simulink model "UIO_example"  (R2019b)
settings: Solver=VariableStepAuto  StartTime=0.0  StopTime=30  RelTol=1e-3
values from neighbouring files (symbols this model uses):
  A = [0 1;-5+Lx -4+epsilon*Lx]    [DAC_UIO_Comp.m]    (also in LinearND_QUANTUM_2020_11_14_2.m = A+(basis{i}*rand()); UIO_adaptive_example.m = [-2379.2 0 0 0 0;0 -2.3 0 0.21 0; UIO_adaptive_example_2.m = [-1/Ta, (alpha+sigma2*wb2)/Ta, (-kb*sigma2*wb2)/Ta, -kb*sigm; UIO_adaptive_example_EEG_Balas_2ch.m)
  B1 = [0;0;0;kq*wa^2]    [UIO_adaptive_example.m]    (also in UIO_adaptive_example_2.m)
  B2 = [68245 0 0;0 -2 0;0 0 2;0 232.75 0; 0 0 -232.75]    [UIO_adaptive_example.m]    (also in UIO_adaptive_example_2.m = [1;0;1;0]; UIO_adaptive_example_EEG.m = ones(opt_order,1); UIO_adaptive_example_EEG_Balas_2ch.m = ones(opt_order,1); UIO_adaptive_example_EEG_ch2.m = ones(opt_order,1))
  C = [1, epsilon]    [DAC_UIO_Comp.m]    (also in UIO_adaptive_example.m = [1 0 0 0 0;0 0 0 1 0; 0 0 0 0 1]; UIO_adaptive_example_2.m = [1 0 0 0;0 1 0 0]; UIO_adaptive_example_EEG_Balas_2ch.m; UIO_adaptive_example_alternative_EEG_ch6.m = ss_c.C)
  F = B2'*P/(C)    [UIO_adaptive_example_2.m]    (also in UIO_adaptive_example_EEG.m = B2'*P/(C_data{opt_order}); UIO_adaptive_example_EEG_ch2.m = B2'*P/(C_data{opt_order}); UIO_adaptive_example_EEG_ch2_DEAP.m = B2'*P/(C_data{opt_order}); UIO_adaptive_example_EEG_ch2_ECEO.m = B2'*P/(C_data{opt_order}))
  Gamma = 20    [UIO_adaptive_example_2.m]    (also in UIO_adaptive_example_EEG.m = 0.001; UIO_adaptive_example_EEG_ch2.m = loop(i); UIO_adaptive_example_EEG_ch2_DEAP.m = loop(i); UIO_adaptive_example_EEG_ch2_ECEO.m = loop(i))
  L = inv(P)*Y    [UIO_adaptive_example.m]    (also in UIO_adaptive_example_2.m; UIO_adaptive_example_EEG.m; UIO_adaptive_example_EEG_ch2.m; UIO_adaptive_example_EEG_ch2_DEAP.m)
settings Model: Creator=Tris  LastModifiedBy=Tris

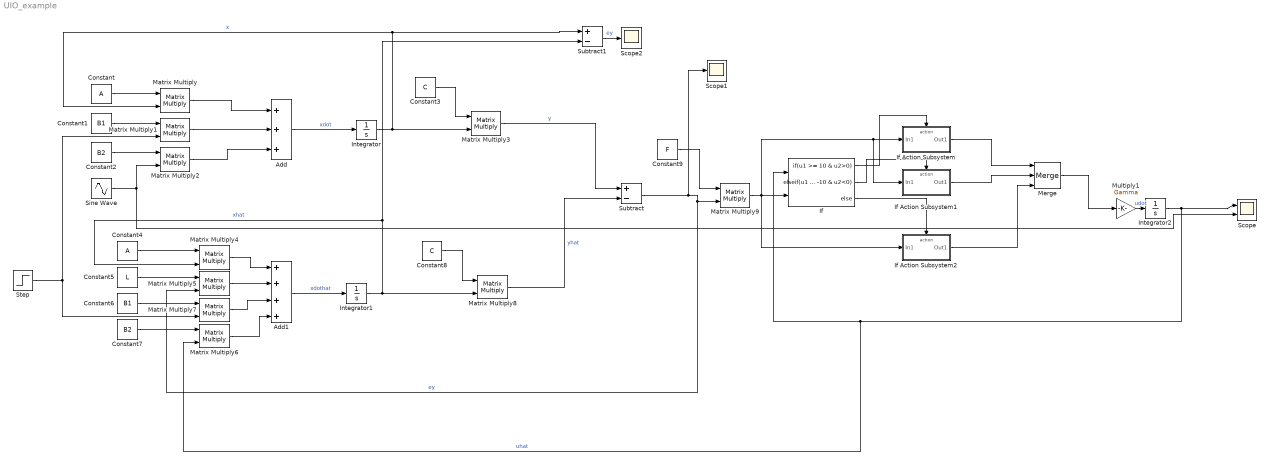
== system UIO_example ==
  Add : Sum  Inputs=+++
  Add1 : Sum  Inputs=++++
  Constant : Constant  Value=A  VectorParams1D=off
  Constant1 : Constant  Value=B1  VectorParams1D=off
  Constant2 : Constant  Value=B2  VectorParams1D=off
  Constant3 : Constant  Value=C  VectorParams1D=off
  Constant4 : Constant  Value=A  VectorParams1D=off
  Constant5 : Constant  Value=L  VectorParams1D=off
  Constant6 : Constant  Value=B1  VectorParams1D=off
  Constant7 : Constant  Value=B2  VectorParams1D=off
  Constant8 : Constant  Value=C  VectorParams1D=off
  Constant9 : Constant  Value=F  VectorParams1D=off
  If : If  NumInputs=2  IfExpression=u1 >= 10 & u2>0  ElseIfExpressions=u1 <= -10 & u2<0
  If Action Subsystem : Subsystem  TreatAsAtomicUnit=on
  If Action Subsystem1 : Subsystem  TreatAsAtomicUnit=on
  If Action Subsystem2 : Subsystem  TreatAsAtomicUnit=on
  Integrator : Integrator  InitialCondition=[1;2;1;2]
  Integrator1 : Integrator
  Integrator2 : Integrator
  Matrix Multiply{,1..9} (10 alike) : Product  Multiplication=Matrix(*)
  Merge : Merge  Inputs=3
  Multiply1 : Gain  Gain=Gamma
  Scope : Scope  NumInputPorts=2
  Scope1 : Scope
  Scope2 : Scope
  Sine Wave : Sin  Amplitude=2  Frequency=2  SampleTime=0
  Step : Step  After=0  SampleTime=0
  Subtract : Sum  Inputs=+-
  Subtract1 : Sum  Inputs=+-
  wires:
  Matrix Multiply/1 -> Add/1
  Constant/1 -> Matrix Multiply/1
  Add/1 -> Integrator/1  "xdot"
  Integrator/1 -> Matrix Multiply3/2, Matrix Multiply/2, Subtract1/1  "x"
  Matrix Multiply1/1 -> Add/2
  Matrix Multiply2/1 -> Add/3
  Constant1/1 -> Matrix Multiply1/1
  Constant2/1 -> Matrix Multiply2/1
  Matrix Multiply3/1 -> Subtract/1  "y"
  Matrix Multiply5/1 -> Add1/2
  Matrix Multiply4/1 -> Add1/1
  Matrix Multiply7/1 -> Add1/3
  Matrix Multiply6/1 -> Add1/4
  Constant4/1 -> Matrix Multiply4/1
  Constant5/1 -> Matrix Multiply5/1
  Constant6/1 -> Matrix Multiply7/1
  Constant7/1 -> Matrix Multiply6/1
  Add1/1 -> Integrator1/1  "xdothat"
  Integrator1/1 -> Matrix Multiply8/2, Subtract1/2, Matrix Multiply4/2  "xhat"
  Matrix Multiply8/1 -> Subtract/2  "yhat"
  Subtract/1 -> Scope1/1, Matrix Multiply5/2, Matrix Multiply9/2  "ey"
  Matrix Multiply9/1 -> If/2, If Action Subsystem2/1(In1), If Action Subsystem1/1(In1), If Action Subsystem/1(In1)
  Integrator2/1 -> Scope/1, Matrix Multiply6/2, If/1  "uhat"
  Step/1 -> Matrix Multiply1/2, Matrix Multiply7/2
  Sine Wave/1 -> Matrix Multiply2/2, Scope/2
  Constant8/1 -> Matrix Multiply8/1
  Constant3/1 -> Matrix Multiply3/1
  Constant9/1 -> Matrix Multiply9/1
  Subtract1/1 -> Scope2/1  "ey"
  Multiply1/1 -> Integrator2/1  "udot"
  If/1 -> If Action Subsystem/Action
  If/2 -> If Action Subsystem1/Action
  If/3 -> If Action Subsystem2/Action
  If Action Subsystem1/1(Out1) -> Merge/2
  If Action Subsystem2/1(Out1) -> Merge/3
  Merge/1 -> Multiply1/1
  If Action Subsystem/1(Out1) -> Merge/1

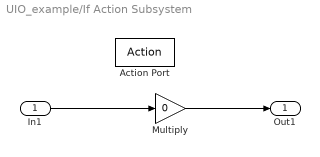
== system UIO_example/If Action Subsystem ==
  In1 : Inport
  Action Port : ActionPort  ActionPortLabel=if(u1 >= 10 & u2>0)
  Multiply : Gain  Gain=0
  Out1 : Outport
  wires:
  In1/1 -> Multiply/1
  Multiply/1 -> Out1/1

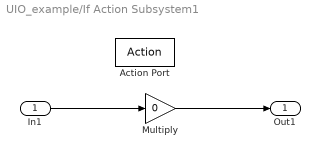
== system UIO_example/If Action Subsystem1 ==
  In1 : Inport
  Action Port : ActionPort  ActionPortLabel=elseif(u1 <= -10 & u2<0)
  Multiply : Gain  Gain=0
  Out1 : Outport
  wires:
  In1/1 -> Multiply/1
  Multiply/1 -> Out1/1

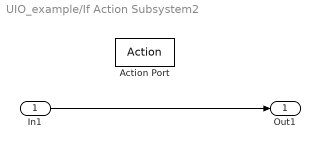
== system UIO_example/If Action Subsystem2 ==
  In1 : Inport
  Action Port : ActionPort  ActionPortLabel=else
  Out1 : Outport
  wires:
  In1/1 -> Out1/1
